simulink model "robot"  (R2016b)
settings: Solver=FixedStepAuto  StartTime=0.0  StopTime=60  FixedStep=0.001  RelTol=1e-3
libraries: fuzblock x1
settings Model: Creator=Truc  LastModifiedBy=Truc

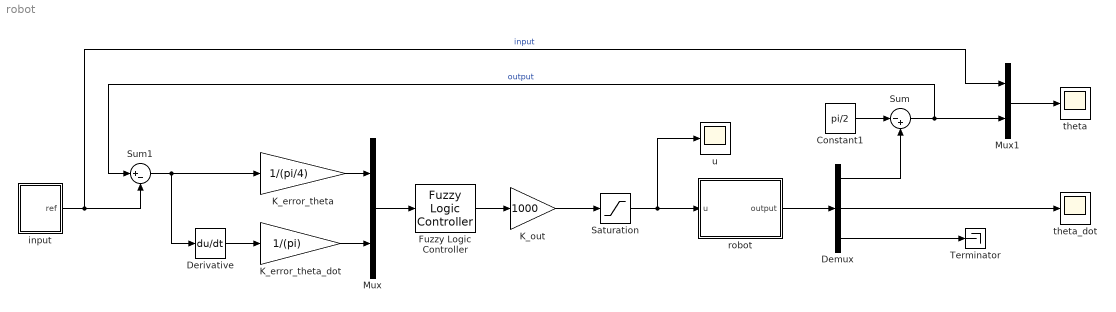
== system robot ==
  Constant1 : Constant  Value=pi/2
  Demux : Demux  Outputs=3
  Derivative : Derivative
  Fuzzy Logic Controller : fuzblock/Fuzzy Logic  Controller  fis='RobotPDFuzzy.fis'
  K_error_theta : Gain  Gain=1/(pi/4)
  K_error_theta_dot : Gain  Gain=1/(pi)
  K_out : Gain  Gain=1000
  Mux : Mux  Inputs=2
  Mux1 : Mux  Inputs=2
  Saturation : Saturate  UpperLimit=50  LowerLimit=-50
  Sum : Sum  Inputs=|-+
  Sum1 : Sum  Inputs=|+-
  Terminator : Terminator
  input : Subsystem
  robot : Subsystem  mask{J=0.015, m=0.15, l=0.5, M_=0.4, lc=0.25, g=9.81, B=0.005, init_theta=0, init_theta_dot=0}
      mask prompts: M_ "M"
  theta : Scope
  theta_dot : Scope
  u : Scope
  wires:
  robot/1(output) -> Demux/1
  Mux/1 -> Fuzzy Logic Controller/1
  Sum1/1 -> K_error_theta/1, Derivative/1
  Derivative/1 -> K_error_theta_dot/1
  Demux/2 -> theta_dot/1
  Sum/1 -> Mux1/2, Sum1/1  "output"
  Demux/3 -> Terminator/1
  input/1(ref) -> Sum1/2, Mux1/1  "input"
  Mux1/1 -> theta/1
  Constant1/1 -> Sum/1
  Demux/1 -> Sum/2
  K_error_theta/1 -> Mux/1
  K_error_theta_dot/1 -> Mux/2
  Fuzzy Logic Controller/1 -> K_out/1
  K_out/1 -> Saturation/1
  Saturation/1 -> u/1, robot/1(u)

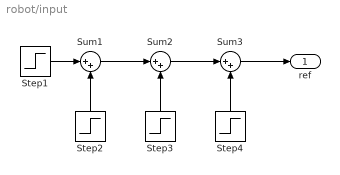
== system robot/input ==
  Step1 : Step  Time=0  After=0  SampleTime=0
  Step2 : Step  Time=15  After=-pi/4  SampleTime=0
  Step3 : Step  Time=30  After=pi/2  SampleTime=0
  Step4 : Step  Time=45  After=-pi/4 - pi/6  SampleTime=0
  Sum1 : Sum  Inputs=|++  SaturateOnIntegerOverflow=on
  Sum2 : Sum  Inputs=|++  SaturateOnIntegerOverflow=on
  Sum3 : Sum  Inputs=|++  SaturateOnIntegerOverflow=on
  ref : Outport
  wires:
  Sum3/1 -> ref/1
  Step4/1 -> Sum3/2
  Sum2/1 -> Sum3/1
  Step3/1 -> Sum2/2
  Step1/1 -> Sum1/1
  Step2/1 -> Sum1/2
  Sum1/1 -> Sum2/1

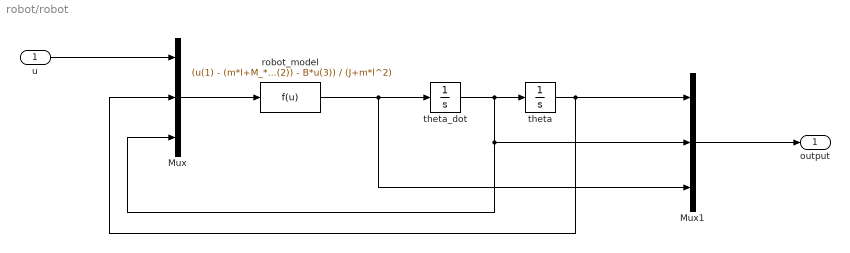
== system robot/robot ==
  u : Inport
  Mux : Mux  Inputs=3
  Mux1 : Mux  Inputs=3
  robot_model : Fcn  Expr=(u(1) - (m*l+M_*lc)*g*cos(u(2)) - B*u(3)) / (J+m*l^2)
  theta : Integrator  InitialCondition=init_theta
  theta_dot : Integrator  InitialCondition=init_theta_dot
  output : Outport
  wires:
  theta/1 -> Mux/2, Mux1/1
  theta_dot/1 -> Mux/3, Mux1/2, theta/1
  Mux1/1 -> output/1
  robot_model/1 -> Mux1/3, theta_dot/1
  Mux/1 -> robot_model/1
  u/1 -> Mux/1
